simulink model "sixDoF_th"  (R2020a)
settings: Solver=VariableStepAuto  StartTime=0.0  StopTime=10.0  RelTol=1e-3
libraries: shared6dof x1, sixDoF_ul x1
settings Model: Creator=Ayaz  LastModifiedBy=Ayaz

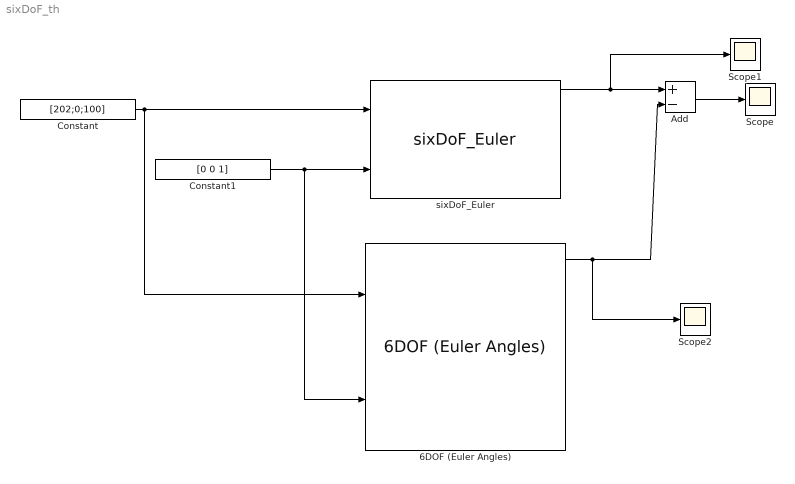
== system sixDoF_th ==
  6DOF (Euler Angles) : shared6dof/6DOF (Euler Angles)  units=Metric (MKS)  mtype=Fixed  rep=Euler Angles  xme_0=[0 0 0]  Vm_0=[0 0 0]  eul_0=[0 0 0]  pm_0=[0 0 0]  mass_0=1.0  mass_e=0.5  mass_f=2.0  inertia=eye(3)  inertia_e=eye(3)  inertia_f=2*eye(3)  k_quat=1.0  vre_flag=on  abi_flag=off  aMode=aMode  xme_statename=''  Vm_statename=''  eul_statename=''  quat_statename=''  pm_statename=''  mass_statename=''
      settings: SourceProductBaseCode=AE,PW,MT,VE,VP
  Add : Sum  Inputs=+-
  Constant : Constant  Value=[202;0;100]
  Constant1 : Constant  Value=[0 0 1]
  Scope : Scope
  Scope1 : Scope
  Scope2 : Scope
  sixDoF_Euler : sixDoF_ul/sixDoF_Euler  mass=1  Jmat=eye(3)  init_O_vKite=[0 0 0]  init_O_rKite=[0 0 0]  init_OwB=[0 0 0]  init_Euler=[0 0 0]
  wires:
  Constant/1 -> 6DOF (Euler Angles)/1, sixDoF_Euler/1
  Constant1/1 -> 6DOF (Euler Angles)/2, sixDoF_Euler/2
  sixDoF_Euler/1 -> Scope1/1, Add/1
  6DOF (Euler Angles)/1 -> Add/2, Scope2/1
  Add/1 -> Scope/1
